simulink library "lib_cart_to_polar_coor_transformer"  (R2023a)
settings: Solver=VariableStepAuto  StartTime=0.0  StopTime=10.0  RelTol=1e-3
libraries: simulink x5, lib_conversion x4, lib_magnitude_calculator x1, lib_dynamic_saturator x1
settings Model: Creator=cav2ofo  LastModifiedBy=xiaoqiang.yuan
settings OptimizationCC: ReuseModelBlockBuffer=off

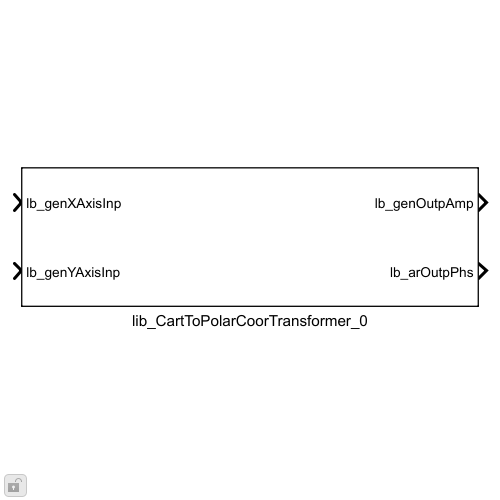
[thumbnail: Simulink's stored preview of the top-level diagram]
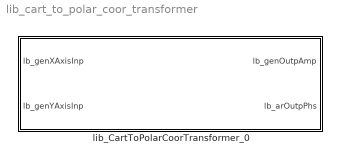
== system lib_cart_to_polar_coor_transformer ==
  lib_CartToPolarCoorTransformer_0 : Subsystem  mask{lb_parAsinLktSize=4095, lb_parAmpLktSize=512, lb_parOutpAmpDataType=fixdt(0,16,2^-10,0)}
      mask prompts: lb_parAsinLktSize "Arcsine function lookup table size:"; lb_parAmpLktSize "Amplitude lookup table size:"; lb_parOutpAmpDataType "Output amplitude data type:"
      mask init:
      | lb_parAsinLktSizeNum = str2double(lb_parAsinLktSize);
      | 
      | data_temp = linspace(0,1,(lb_parAsinLktSizeNum+1)/2);
      | lb_parAsinFunLkt = asin([flip(-data_temp(2:end)) data_temp]);
      | 
      | % Warning suppression due to intentional overflow wrapping
      | Simulink.suppressDiagnostic([gcb,'/sss_PhaseAngleCalculator/ias_NonZeroInput/Data Type Conversion2'],...
      |  'SimulinkFixedPoint:util:Overflowoccurred');
      | Simulink.suppressDiagnostic([gcb,'/sss_PhaseAngleCalculator/ias_NonZeroInput/sss_AsinFunctionCorrector/ias_AngleShiftApplied/Add'],...
      |  'SimulinkFixedPoint:util:Overflowoccurred');
      mask TypeOptions lb_parAsinLktSize: 1023 | 2047 | 4095 | 8191 | 16383 | 32767 | 65535
      mask TypeOptions lb_parAmpLktSize: lib_MagnitudeCalculator_1/lb_parLktSize
      mask DialogControl DescGroupVar Prompt: VHIT control library
      mask DialogControl DescTextVar Prompt: Cartesian to polar coordinates transformer
      mask DialogControl Container3 Prompt: Data type

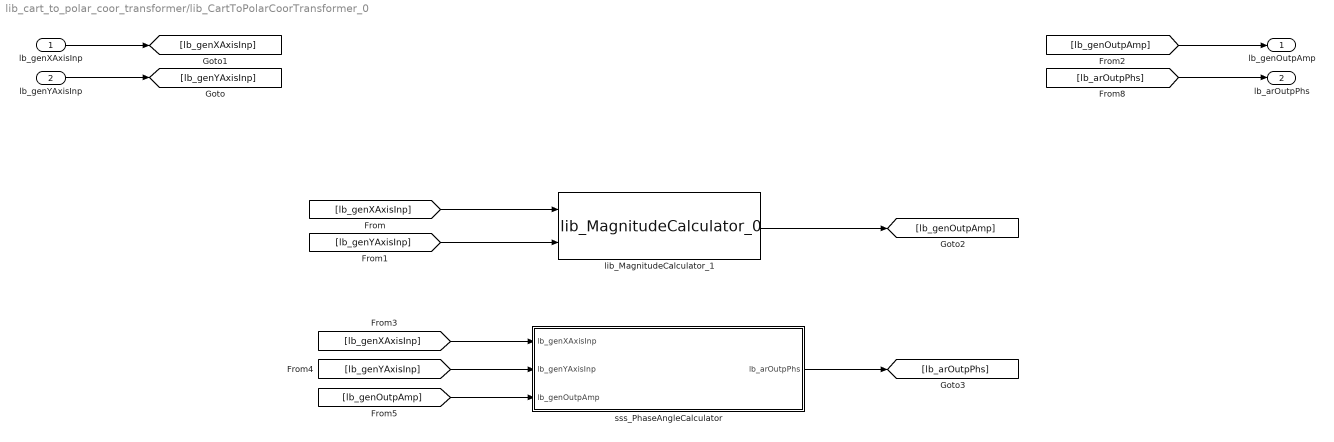
== system lib_cart_to_polar_coor_transformer/lib_CartToPolarCoorTransformer_0 ==
  lb_genXAxisInp : Inport
  lb_genYAxisInp : Inport  Port=2
  lib_MagnitudeCalculator_1 : lib_magnitude_calculator/lib_MagnitudeCalculator_0  lb_parLktSize=512  lb_parOutpDataType=lb_parOutpAmpDataType
  sss_PhaseAngleCalculator : Subsystem
  lb_genOutpAmp : Outport
  lb_arOutpPhs : Outport  Port=2
  wires:
  [lb_genOutpAmp] -> sss_PhaseAngleCalculator/3(lb_genOutpAmp)
  [lb_genYAxisInp] -> sss_PhaseAngleCalculator/2(lb_genYAxisInp)
  [lb_genXAxisInp] -> sss_PhaseAngleCalculator/1(lb_genXAxisInp)
  sss_PhaseAngleCalculator/1(lb_arOutpPhs) -> [lb_arOutpPhs]
  [lb_arOutpPhs] -> lb_arOutpPhs/1
  [lb_genOutpAmp] -> lb_genOutpAmp/1
  lb_genXAxisInp/1 -> [lb_genXAxisInp]
  lb_genYAxisInp/1 -> [lb_genYAxisInp]
  [lb_genXAxisInp] -> lib_MagnitudeCalculator_1/1
  [lb_genYAxisInp] -> lib_MagnitudeCalculator_1/2
  lib_MagnitudeCalculator_1/1 -> [lb_genOutpAmp]

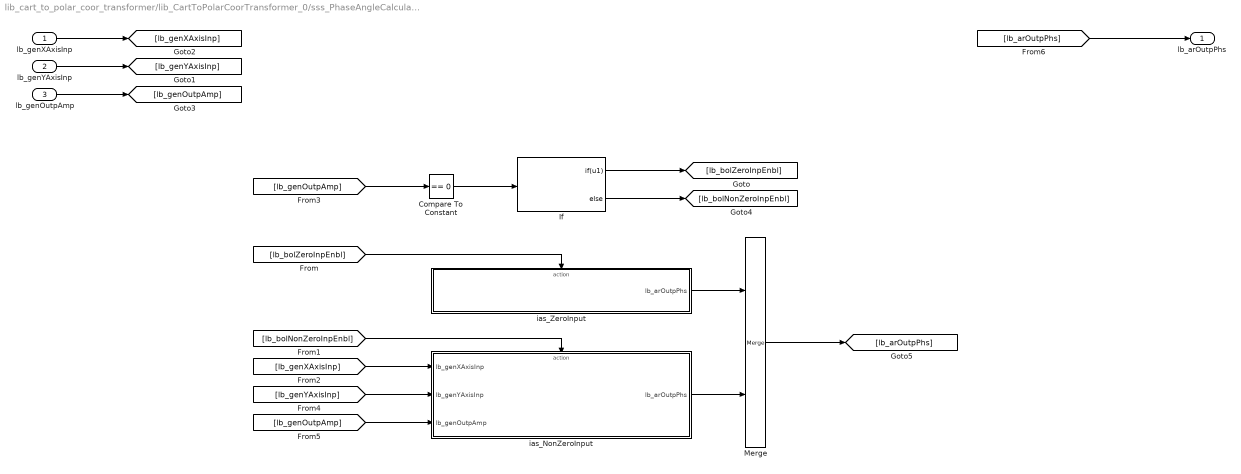
== system lib_cart_to_polar_coor_transformer/lib_CartToPolarCoorTransformer_0/sss_PhaseAngleCalculator ==
  lb_genXAxisInp : Inport
  lb_genYAxisInp : Inport  Port=2
  lb_genOutpAmp : Inport  Port=3
  Compare To Constant : simulink/Logic and Bit Operations/Compare To Constant  relop===  const=0  OutDataTypeStr=boolean
  If : If  IfExpression=u1
  Merge : Merge
  ias_NonZeroInput : Subsystem  TreatAsAtomicUnit=on
      settings: RTWSystemCode=Inline
  ias_ZeroInput : Subsystem  TreatAsAtomicUnit=on
      settings: RTWSystemCode=Inline
  lb_arOutpPhs : Outport
  wires:
  [lb_arOutpPhs] -> lb_arOutpPhs/1
  Merge/1 -> [lb_arOutpPhs]
  ias_NonZeroInput/1(lb_arOutpPhs) -> Merge/2
  ias_ZeroInput/1(lb_arOutpPhs) -> Merge/1
  [lb_genYAxisInp] -> ias_NonZeroInput/2(lb_genYAxisInp)
  [lb_genOutpAmp] -> ias_NonZeroInput/3(lb_genOutpAmp)
  [lb_genXAxisInp] -> ias_NonZeroInput/1(lb_genXAxisInp)
  lb_genYAxisInp/1 -> [lb_genYAxisInp]
  lb_genXAxisInp/1 -> [lb_genXAxisInp]
  lb_genOutpAmp/1 -> [lb_genOutpAmp]
  [lb_bolNonZeroInpEnbl] -> ias_NonZeroInput/Action
  [lb_bolZeroInpEnbl] -> ias_ZeroInput/Action
  If/1 -> [lb_bolZeroInpEnbl]
  If/2 -> [lb_bolNonZeroInpEnbl]
  Compare To Constant/1 -> If/1
  [lb_genOutpAmp] -> Compare To Constant/1

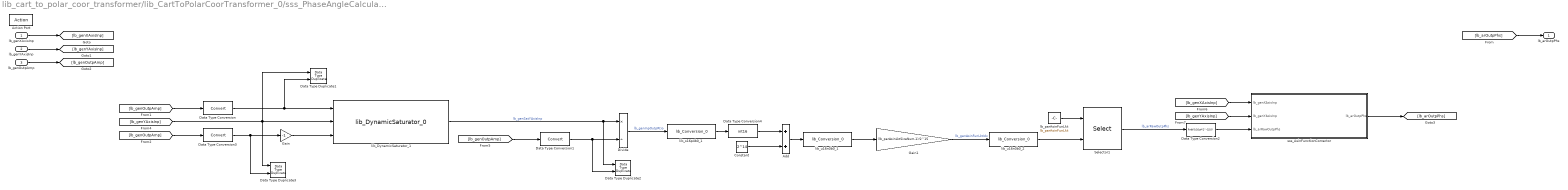
== system lib_cart_to_polar_coor_transformer/lib_CartToPolarCoorTransformer_0/sss_PhaseAngleCalculator/ias_NonZeroInput ==
  lb_genXAxisInp : Inport
  lb_genYAxisInp : Inport  Port=2
  lb_genOutpAmp : Inport  Port=3
  Action Port : ActionPort
  Add : Sum  OutDataTypeStr=Inherit: Inherit via back propagation  RndMeth=Simplest
  Constant : Constant  Value=2^14  OutDataTypeStr=uint16
  Data Type Duplicate1 : DataTypeDuplicate
  Data Type Duplicate2 : DataTypeDuplicate
  Data Type Duplicate3 : DataTypeDuplicate
  Data Type Conversion : DataTypeConversion  SaturateOnIntegerOverflow=off  RndMeth=Floor
  Data Type Conversion1 : DataTypeConversion  SaturateOnIntegerOverflow=off  RndMeth=Floor
  Data Type Conversion2 : DataTypeConversion  OutDataTypeStr=fixdt(0,16,pi*2^-15,0)  SaturateOnIntegerOverflow=off  RndMeth=Floor
  Data Type Conversion3 : DataTypeConversion  SaturateOnIntegerOverflow=off  RndMeth=Floor
  Data Type Conversion4 : DataTypeConversion  OutDataTypeStr=int16  ConvertRealWorld=Stored Integer (SI)  RndMeth=Simplest  SaturateOnIntegerOverflow=off
  Divide : Product  Inputs=*/  OutDataTypeStr=Inherit: Inherit via back propagation  RndMeth=Simplest
  Gain : Gain  Gain=-1  RndMeth=Simplest  OutDataTypeStr=Inherit: Same as input
  Gain1 : Gain  Gain=(lb_parAsinLktSizeNum-1)/2^15  OutDataTypeStr=uint16  RndMeth=Simplest
  Selector1 : Selector  IndexMode=Zero-based  InputPortWidth=lb_parAsinLktSizeNum  IndexOptions=Index vector (port)  Indices=[1 3]  OutputSizes=1
  lb_parAsinFunLkt : Constant  Value=lb_parAsinFunLkt  OutDataTypeStr=fixdt(1,16,pi*2^-15,0)
  lib_DynamicSaturator_1 : lib_dynamic_saturator/lib_DynamicSaturator_0
  lib_s16p4b0_1 : lib_conversion/lib_Conversion_0  lb_parDataType=fixdt(1,16,2^-14,0)  lb_parOutpMaxVal=[]  lb_parOutpMinVal=[]  lb_parSatFlag=off
  lib_u16n0b0_1 : lib_conversion/lib_Conversion_0  lb_parDataType=uint16  lb_parOutpMaxVal=[]  lb_parOutpMinVal=[]  lb_parSatFlag=off
  lib_u16n0b0_2 : lib_conversion/lib_Conversion_0  lb_parDataType=uint16  lb_parOutpMaxVal=[]  lb_parOutpMinVal=[]  lb_parSatFlag=off
  sss_AsinFunctionCorrector : Subsystem
  lb_arOutpPhs : Outport
  wires:
  Data Type Conversion2/1 -> sss_AsinFunctionCorrector/3(lb_arRawOutpPhs)
  [lb_arOutpPhs] -> lb_arOutpPhs/1
  sss_AsinFunctionCorrector/1(lb_arOutpPhs) -> [lb_arOutpPhs]
  lb_genOutpAmp/1 -> [lb_genOutpAmp]
  lb_genYAxisInp/1 -> [lb_genYAxisInp]
  lb_genXAxisInp/1 -> [lb_genXAxisInp]
  [lb_genXAxisInp] -> sss_AsinFunctionCorrector/1(lb_genXAxisInp)
  [lb_genYAxisInp] -> sss_AsinFunctionCorrector/2(lb_genYAxisInp)
  [lb_genOutpAmp] -> Data Type Conversion1/1
  Divide/1 -> lib_s16p4b0_1/1  "lb_genInpOutpRtio"
  [lb_genYAxisInp] -> lib_DynamicSaturator_1/2, Data Type Duplicate1/1, Data Type Duplicate3/1
  [lb_genOutpAmp] -> Data Type Conversion/1
  Data Type Conversion3/1 -> Data Type Duplicate3/2, Gain/1
  Data Type Conversion/1 -> lib_DynamicSaturator_1/1, Data Type Duplicate1/2
  lib_DynamicSaturator_1/1 -> Data Type Duplicate2/1, Divide/1  "lb_genSatYAxisInp"
  Data Type Conversion1/1 -> Data Type Duplicate2/2, Divide/2
  Selector1/1 -> Data Type Conversion2/1  "lb_arRawOutpPhs"
  [lb_genOutpAmp] -> Data Type Conversion3/1
  Gain/1 -> lib_DynamicSaturator_1/3
  Data Type Conversion4/1 -> Add/1
  Constant/1 -> Add/2
  Add/1 -> lib_u16n0b0_1/1
  lb_parAsinFunLkt/1 -> Selector1/1
  lib_s16p4b0_1/1 -> Data Type Conversion4/1
  Gain1/1 -> lib_u16n0b0_2/1  "lb_genAsinFunLktIdx"
  lib_u16n0b0_1/1 -> Gain1/1
  lib_u16n0b0_2/1 -> Selector1/2

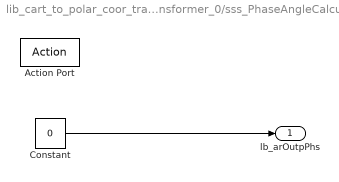
== system lib_cart_to_polar_coor_transformer/lib_CartToPolarCoorTransformer_0/sss_PhaseAngleCalculator/ias_ZeroInput ==
  Action Port : ActionPort
  Constant : Constant  Value=0  OutDataTypeStr=fixdt(0,16,pi*2^-15,0)
  lb_arOutpPhs : Outport
  wires:
  Constant/1 -> lb_arOutpPhs/1

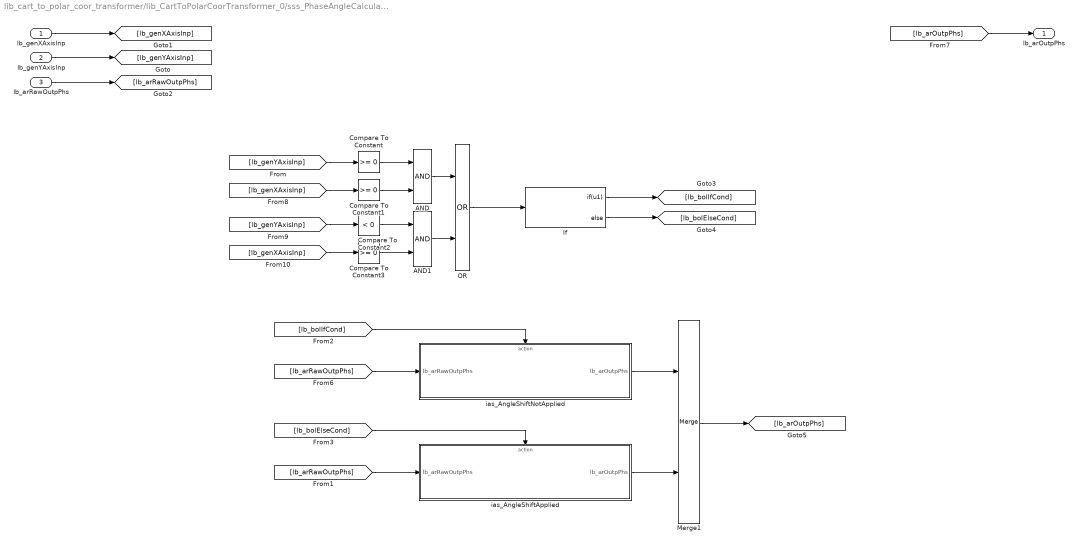
== system lib_cart_to_polar_coor_transformer/lib_CartToPolarCoorTransformer_0/sss_PhaseAngleCalculator/ias_NonZeroInput/sss_AsinFunctionCorrector ==
  lb_genXAxisInp : Inport
  lb_genYAxisInp : Inport  Port=2
  lb_arRawOutpPhs : Inport  Port=3
  AND : Logic  AllPortsSameDT=off  OutDataTypeStr=boolean
  AND1 : Logic  AllPortsSameDT=off  OutDataTypeStr=boolean
  Compare To Constant : simulink/Logic and Bit Operations/Compare To Constant  relop=>=  const=0  OutDataTypeStr=boolean
  Compare To Constant1 : simulink/Logic and Bit Operations/Compare To Constant  relop=>=  const=0  OutDataTypeStr=boolean
  Compare To Constant2 : simulink/Logic and Bit Operations/Compare To Constant  relop=<  const=0  OutDataTypeStr=boolean
  Compare To Constant3 : simulink/Logic and Bit Operations/Compare To Constant  relop=>=  const=0  OutDataTypeStr=boolean
  If : If  IfExpression=u1
  Merge1 : Merge
  OR : Logic  Operator=OR  AllPortsSameDT=off  OutDataTypeStr=boolean
  ias_AngleShiftApplied : Subsystem  TreatAsAtomicUnit=on
  ias_AngleShiftNotApplied : Subsystem  TreatAsAtomicUnit=on
  lb_arOutpPhs : Outport
  wires:
  [lb_arRawOutpPhs] -> ias_AngleShiftApplied/1(lb_arRawOutpPhs)
  [lb_arOutpPhs] -> lb_arOutpPhs/1
  Merge1/1 -> [lb_arOutpPhs]
  ias_AngleShiftNotApplied/1(lb_arOutpPhs) -> Merge1/1
  ias_AngleShiftApplied/1(lb_arOutpPhs) -> Merge1/2
  [lb_arRawOutpPhs] -> ias_AngleShiftNotApplied/1(lb_arRawOutpPhs)
  [lb_bolElseCond] -> ias_AngleShiftApplied/Action
  If/2 -> [lb_bolElseCond]
  [lb_bolIfCond] -> ias_AngleShiftNotApplied/Action
  If/1 -> [lb_bolIfCond]
  [lb_genYAxisInp] -> Compare To Constant/1
  lb_arRawOutpPhs/1 -> [lb_arRawOutpPhs]
  lb_genYAxisInp/1 -> [lb_genYAxisInp]
  lb_genXAxisInp/1 -> [lb_genXAxisInp]
  Compare To Constant/1 -> AND/1
  [lb_genXAxisInp] -> Compare To Constant1/1
  Compare To Constant1/1 -> AND/2
  [lb_genYAxisInp] -> Compare To Constant2/1
  [lb_genXAxisInp] -> Compare To Constant3/1
  Compare To Constant3/1 -> AND1/2
  Compare To Constant2/1 -> AND1/1
  OR/1 -> If/1
  AND1/1 -> OR/2
  AND/1 -> OR/1

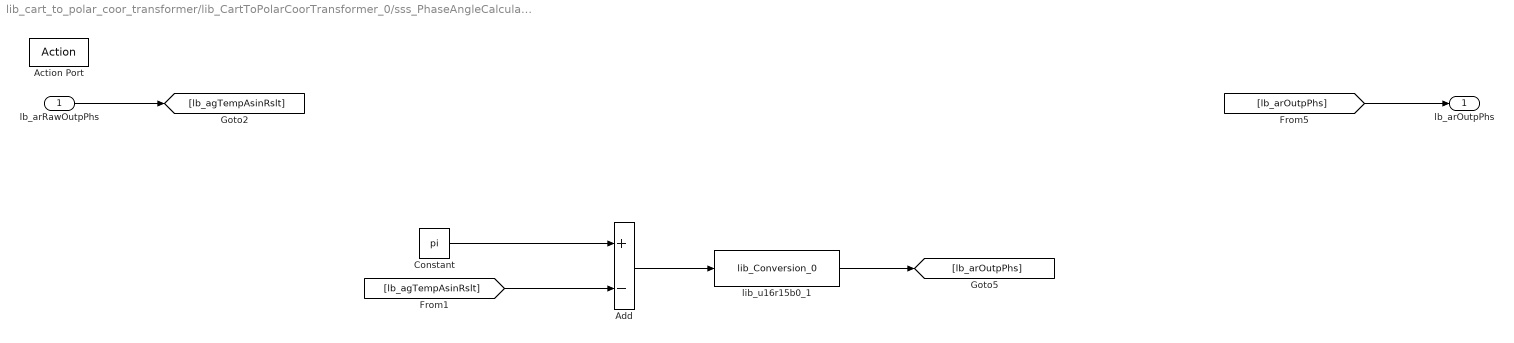
== system lib_cart_to_polar_coor_transformer/lib_CartToPolarCoorTransformer_0/sss_PhaseAngleCalculator/ias_NonZeroInput/sss_AsinFunctionCorrector/ias_AngleShiftApplied ==
  lb_arRawOutpPhs : Inport
  Action Port : ActionPort
  Add : Sum  Inputs=+-  OutDataTypeStr=Inherit: Inherit via back propagation  RndMeth=Simplest
  Constant : Constant  Value=pi  OutDataTypeStr=fixdt(0,16,pi*2^-15,0)
  lib_u16r15b0_1 : lib_conversion/lib_Conversion_0  lb_parDataType=fixdt(0,16,pi*2^-15,0)  lb_parOutpMaxVal=[]  lb_parOutpMinVal=[]  lb_parSatFlag=off
  lb_arOutpPhs : Outport
  wires:
  lb_arRawOutpPhs/1 -> [lb_agTempAsinRslt]
  [lb_arOutpPhs] -> lb_arOutpPhs/1
  Add/1 -> lib_u16r15b0_1/1
  lib_u16r15b0_1/1 -> [lb_arOutpPhs]
  [lb_agTempAsinRslt] -> Add/2
  Constant/1 -> Add/1

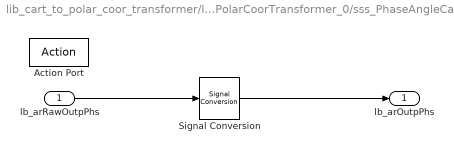
== system lib_cart_to_polar_coor_transformer/lib_CartToPolarCoorTransformer_0/sss_PhaseAngleCalculator/ias_NonZeroInput/sss_AsinFunctionCorrector/ias_AngleShiftNotApplied ==
  lb_arRawOutpPhs : Inport
  Action Port : ActionPort
  Signal Conversion : SignalConversion  OverrideOpt=off
  lb_arOutpPhs : Outport
  wires:
  lb_arRawOutpPhs/1 -> Signal Conversion/1
  Signal Conversion/1 -> lb_arOutpPhs/1
